simulink model "my_gm_HDLModulatorFull"  (R2024a)
settings: Solver=FixedStepDiscrete  StartTime=0.0  StopTime=stopTime  RelTol=1e-3
values from neighbouring files (symbols this model uses):
  dataSymbols = [ ... (first row only)    [testModulatorFull.m]
undefined symbols (not defined in the file or in its folder): fPHY, fs, interpolatorFilter, numDataCarriers
libraries: dspsigops x56, hdlmdlgenlib x56, hdlsllib x8, dspsrcs4 x4, commdigbbndam3 x2, whdlutilities x1, commdigbbndpm3 x1, dsphdlsigops2 x1, dsphdlfiltering2 x1, whdlmod x1, HDL_ieee_8021513 x1
(part 1 of 2)
settings Model: SimulationMode=accelerator  Creator=cotti  LastModifiedBy=cotti
settings OptimizationCC: BlockReduction=off  ConditionallyExecuteInputs=off  DefaultParameterBehavior=Inlined  InheritOutputTypeSmallerThanSingle=on
settings DebuggingCC: AlgebraicLoopMsg=error  ArtificialAlgebraicLoopMsg=none  InheritedTsInSrcMsg=none  SingleTaskRateTransMsg=error  UnconnectedInputMsg=warning  UnconnectedOutputMsg=warning  UnconnectedLineMsg=warning
settings HardwareCC: ProdBitPerPointer=32  ProdBitPerSizeT=32  ProdBitPerPtrDiffT=32  ProdLargestAtomicFloat=None  ProdIntDivRoundTo=Undefined  ProdEndianess=Unspecified  ProdWordSize=32  ProdHWDeviceType=ASIC/FPGA->ASIC/FPGA  TargetBitPerLong=64  TargetBitPerPointer=64  TargetBitPerSizeT=64  TargetBitPerPtrDiffT=64  TargetLongLongMode=on  TargetIntDivRoundTo=Zero  TargetEndianess=LittleEndian  TargetWordSize=64  TargetHWDeviceType=Custom Processor->MATLAB Host Computer  ProdEqTarget=off

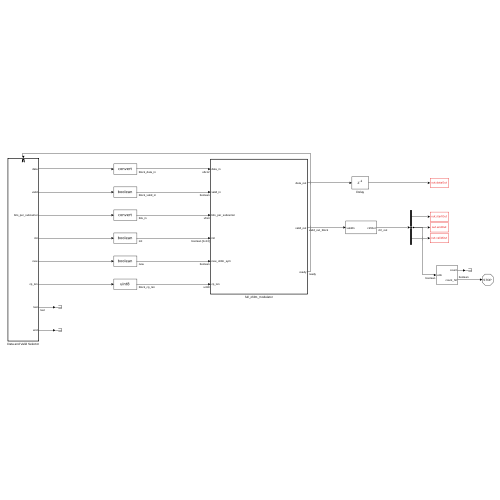
[thumbnail: Simulink's stored preview of the top-level diagram]
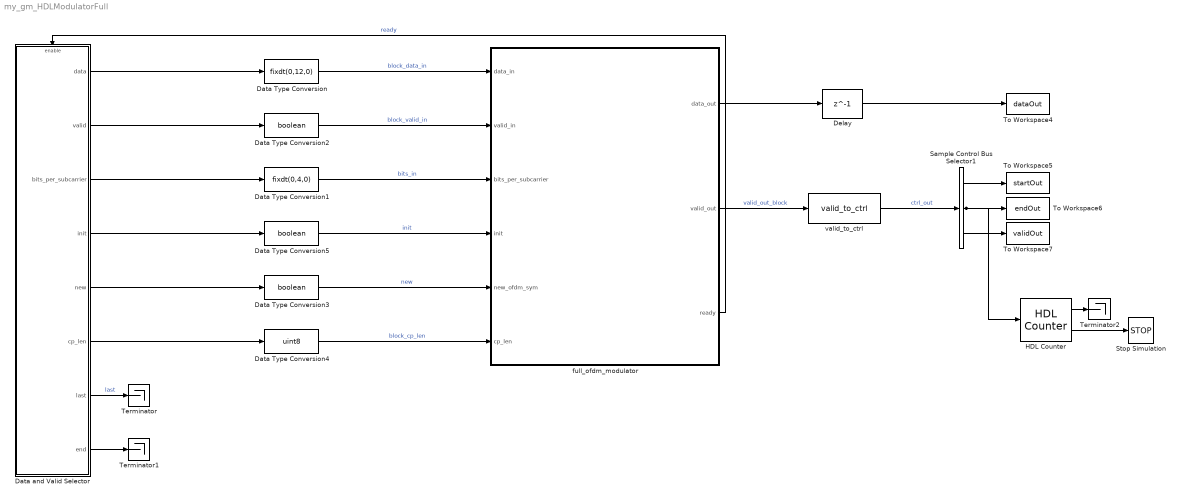
== system my_gm_HDLModulatorFull ==
  Data Type Conversion : DataTypeConversion  OutDataTypeStr=fixdt(0,12,0)  SaturateOnIntegerOverflow=off  RndMeth=Floor  LockScale=on
  Data Type Conversion1 : DataTypeConversion  OutDataTypeStr=fixdt(0,4,0)  SaturateOnIntegerOverflow=off  RndMeth=Floor  LockScale=on
  Data Type Conversion2 : DataTypeConversion  OutDataTypeStr=boolean  SaturateOnIntegerOverflow=off  RndMeth=Floor  LockScale=on
  Data Type Conversion3 : DataTypeConversion  OutDataTypeStr=boolean  SaturateOnIntegerOverflow=off  RndMeth=Floor  LockScale=on
  Data Type Conversion4 : DataTypeConversion  OutDataTypeStr=uint8  SaturateOnIntegerOverflow=off  RndMeth=Floor  LockScale=on
  Data Type Conversion5 : DataTypeConversion  OutDataTypeStr=boolean  SaturateOnIntegerOverflow=off  RndMeth=Floor  LockScale=on
  Data and Valid Selector : Subsystem  TreatAsAtomicUnit=on
  Delay : Delay  DelayLength=1  InitialCondition=0  UseCircularBuffer=on
  HDL Counter : hdlsllib/Sources/HDL Counter  CountType=Count limited  CountInit=0  CountStep=1  CountMax=numberOfRepetitions  CountFromType=Initial value  CountFrom=0  CountResetPort=off  CountLoadPort=off  CountEnbPort=on  CountDirPort=off  CountHitOutputPort=on  CountDataType=Unsigned  CountWordLen=8  CountFracLen=0  CountSampTime=1
  Sample Control Bus Selector1 : whdlutilities/Sample Control Bus Selector  OutputSignals=start,end,valid
  Stop Simulation : Stop
  Terminator : Terminator
  Terminator1 : Terminator
  Terminator2 : Terminator
  To Workspace4 : ToWorkspace  VariableName=dataOut  SampleTime=1/fs
      settings: Save2DSignal=2-D array (concatenate along first dimension)
  To Workspace5 : ToWorkspace  VariableName=startOut  SampleTime=1/fs
      settings: Save2DSignal=2-D array (concatenate along first dimension)
  To Workspace6 : ToWorkspace  VariableName=endOut  SampleTime=1/fs
      settings: Save2DSignal=2-D array (concatenate along first dimension)
  To Workspace7 : ToWorkspace  VariableName=validOut  SampleTime=1/fs
      settings: Save2DSignal=2-D array (concatenate along first dimension)
  full_ofdm_modulator : Subsystem  TreatAsAtomicUnit=on
  valid_to_ctrl : HDL_ieee_8021513/valid_to_ctrl  SystemSampleTime=-1  VariantActivationTime=update diagram  AllowFlexibleInterface=on  Latency=0  AutoFrameSizeCalculation=off
      settings: SourceProductName=HDL IEEE 8021513
  wires:
  HDL Counter/2 -> Stop Simulation/1
  HDL Counter/1 -> Terminator2/1
  Delay/1 -> To Workspace4/1
  full_ofdm_modulator/3(ready) -> Data and Valid Selector/Enable  "ready"
  Data Type Conversion5/1 -> full_ofdm_modulator/4(init)  "init"
  Data Type Conversion3/1 -> full_ofdm_modulator/5(new_ofdm_sym)  "new"
  Data and Valid Selector/7(last) -> Terminator/1  "last"
  Data and Valid Selector/5(new) -> Data Type Conversion3/1
  Data and Valid Selector/3(bits_per_subcarrier) -> Data Type Conversion1/1
  Data and Valid Selector/1(data) -> Data Type Conversion/1
  Data Type Conversion/1 -> full_ofdm_modulator/1(data_in)  "block_data_in"
  Data and Valid Selector/2(valid) -> Data Type Conversion2/1
  Data and Valid Selector/4(init) -> Data Type Conversion5/1
  Data and Valid Selector/6(cp_len) -> Data Type Conversion4/1
  Data Type Conversion4/1 -> full_ofdm_modulator/6(cp_len)  "block_cp_len"
  Data Type Conversion2/1 -> full_ofdm_modulator/2(valid_in)  "block_valid_in"
  Data and Valid Selector/8(end) -> Terminator1/1
  Data Type Conversion1/1 -> full_ofdm_modulator/3(bits_per_subcarrier)  "bits_in"
  Sample Control Bus Selector1/2 -> To Workspace6/1, HDL Counter/1
  Sample Control Bus Selector1/1 -> To Workspace5/1
  valid_to_ctrl/1 -> Sample Control Bus Selector1/1  "ctrl_out"
  Sample Control Bus Selector1/3 -> To Workspace7/1
  full_ofdm_modulator/1(data_out) -> Delay/1
  full_ofdm_modulator/2(valid_out) -> valid_to_ctrl/1  "valid_out_block"

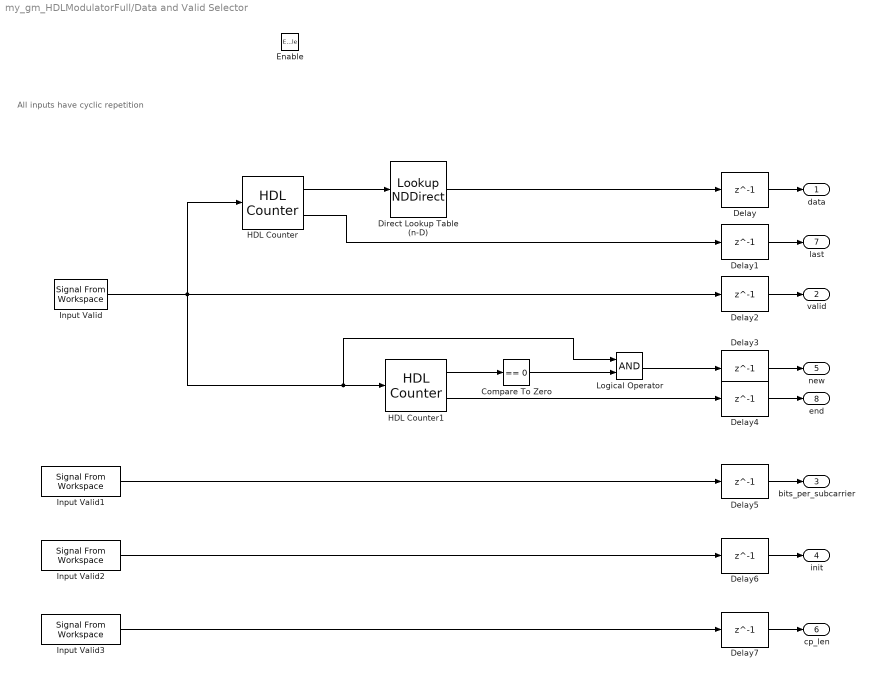
== system my_gm_HDLModulatorFull/Data and Valid Selector ==
  note: All inputs have cyclic repetition
  Enable : EnablePort
  Compare To Zero : hdlsllib/Logic and Bit Operations/Compare To Zero  relop===  OutDataTypeStr=boolean
  Delay{,1..7} (8 alike) : Delay  DelayLength=1  InitialCondition=0  UseCircularBuffer=on
  Direct Lookup Table (n-D) : LookupNDDirect  NumberOfTableDimensions=1  Table=dataSymbols  DiagnosticForOutOfRangeInput=Error  TableDataTypeStr=fixdt(0,12,0)
  HDL Counter : hdlsllib/Sources/HDL Counter  CountType=Count limited  CountInit=0  CountStep=1  CountMax=length(dataSymbols) -1  CountFromType=Initial value  CountFrom=0  CountResetPort=off  CountLoadPort=off  CountEnbPort=on  CountDirPort=off  CountHitOutputPort=on  CountDataType=Unsigned  CountWordLen=nextpow2(length(dataSymbols))  CountFracLen=0  CountSampTime=1
  HDL Counter1 : hdlsllib/Sources/HDL Counter  CountType=Count limited  CountInit=0  CountStep=1  CountMax=numDataCarriers-1  CountFromType=Initial value  CountFrom=0  CountResetPort=off  CountLoadPort=off  CountEnbPort=on  CountDirPort=off  CountHitOutputPort=on  CountDataType=Unsigned  CountWordLen=nextpow2(numDataCarriers)  CountFracLen=0  CountSampTime=1
  Input Valid : dspsrcs4/Signal From Workspace  X=validIn  Ts=1/fPHY  nsamps=1  OutputAfterFinalValue=Cyclic repetition  ignoreOrWarnInputAndFrameLengths=off  OutputFrames=off
  Input Valid1 : dspsrcs4/Signal From Workspace  X=bitsPerSubcarrier  Ts=1/fPHY  nsamps=1  OutputAfterFinalValue=Cyclic repetition  ignoreOrWarnInputAndFrameLengths=off  OutputFrames=off
  Input Valid2 : dspsrcs4/Signal From Workspace  X=init  Ts=1/fPHY  nsamps=1  OutputAfterFinalValue=Cyclic repetition  ignoreOrWarnInputAndFrameLengths=off  OutputFrames=off
  Input Valid3 : dspsrcs4/Signal From Workspace  X=cpLen  Ts=1/fPHY  nsamps=1  OutputAfterFinalValue=Cyclic repetition  ignoreOrWarnInputAndFrameLengths=off  OutputFrames=off
  Logical Operator : Logic  AllPortsSameDT=off  OutDataTypeStr=boolean
  data : Outport  InitialOutput=0  VectorParamsAs1DForOutWhenUnconnected=off
  valid : Outport  Port=2  InitialOutput=0  VectorParamsAs1DForOutWhenUnconnected=off
  bits_per_subcarrier : Outport  Port=3  VectorParamsAs1DForOutWhenUnconnected=off
  init : Outport  Port=4  VectorParamsAs1DForOutWhenUnconnected=off
  new : Outport  Port=5  VectorParamsAs1DForOutWhenUnconnected=off
  cp_len : Outport  Port=6  VectorParamsAs1DForOutWhenUnconnected=off
  last : Outport  Port=7  VectorParamsAs1DForOutWhenUnconnected=off
  end : Outport  Port=8  VectorParamsAs1DForOutWhenUnconnected=off
  wires:
  Delay7/1 -> cp_len/1
  Delay6/1 -> init/1
  Delay5/1 -> bits_per_subcarrier/1
  Delay4/1 -> end/1
  Delay3/1 -> new/1
  Delay2/1 -> valid/1
  Delay1/1 -> last/1
  Delay/1 -> data/1
  Input Valid1/1 -> Delay5/1
  Input Valid2/1 -> Delay6/1
  Input Valid3/1 -> Delay7/1
  Input Valid/1 -> HDL Counter1/1, Logical Operator/1, Delay2/1, HDL Counter/1
  HDL Counter1/2 -> Delay4/1
  Logical Operator/1 -> Delay3/1
  Compare To Zero/1 -> Logical Operator/2
  HDL Counter1/1 -> Compare To Zero/1
  HDL Counter/2 -> Delay1/1
  Direct Lookup Table (n-D)/1 -> Delay/1
  HDL Counter/1 -> Direct Lookup Table (n-D)/1

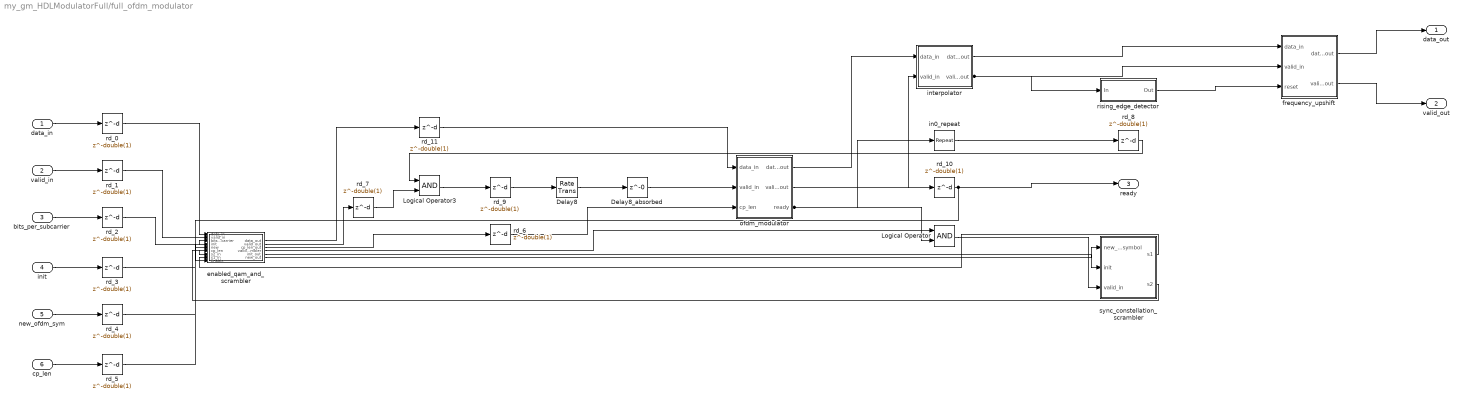
== system my_gm_HDLModulatorFull/full_ofdm_modulator ==
  data_in : Inport  OutDataTypeStr=fixdt(0, 12, 0)  PortDimensions=1  SampleTime=2e-08
  valid_in : Inport  Port=2  OutDataTypeStr=boolean  PortDimensions=1  SampleTime=2e-08
  bits_per_subcarrier : Inport  Port=3  OutDataTypeStr=fixdt(0, 4, 0)  PortDimensions=1  SampleTime=2e-08
  init : Inport  Port=4  OutDataTypeStr=boolean  PortDimensions=[1 13]  SampleTime=2e-08
  new_ofdm_sym : Inport  Port=5  OutDataTypeStr=boolean  PortDimensions=1  SampleTime=2e-08
  cp_len : Inport  Port=6  OutDataTypeStr=uint8  PortDimensions=1  SampleTime=2e-08
  Delay8 : RateTransition  OutPortSampleTimeOpt=Multiple of input port sample time  OutPortSampleTimeMultiple=2
  Delay8_absorbed : Delay  DelayLength=0
  Logical Operator : Logic  AllPortsSameDT=off  OutDataTypeStr=boolean  SampleTime=2e-08
  Logical Operator3 : Logic  AllPortsSameDT=off  OutDataTypeStr=boolean  SampleTime=1e-08
  enabled_qam_and_scrambler : Subsystem
  frequency_upshift : Subsystem
  in0_repeat : dspsigops/Repeat  FactorSource=Dialog parameter  N=double(2)  Nmax=16  RateOptions=Allow multirate processing  ic=0  mode=Unused parameter value
  interpolator : Subsystem
  ofdm_modulator : Subsystem
  rd_{0..6,10..11} (9 alike) : Delay  DelayLength=double(1)  InitialCondition=0  SampleTime=2e-08
  rd_7 : Delay  DelayLength=double(1)  InitialCondition=0  SampleTime=1e-08
  rd_8 : Delay  DelayLength=double(1)  InitialCondition=0  SampleTime=1e-08
  rd_9 : Delay  DelayLength=double(1)  InitialCondition=0  SampleTime=1e-08
  rising_edge_detector : Subsystem
  sync_constellation_scrambler : Subsystem
  data_out : Outport  SampleTime=1e-08  VectorParamsAs1DForOutWhenUnconnected=off
  valid_out : Outport  Port=2  SampleTime=1e-08  VectorParamsAs1DForOutWhenUnconnected=off
  ready : Outport  Port=3  SampleTime=2e-08  VectorParamsAs1DForOutWhenUnconnected=off
  wires:
  data_in/1 -> rd_0/1
  valid_in/1 -> rd_1/1
  bits_per_subcarrier/1 -> rd_2/1
  init/1 -> rd_3/1
  new_ofdm_sym/1 -> rd_4/1
  cp_len/1 -> rd_5/1
  frequency_upshift/1(data_out) -> data_out/1
  frequency_upshift/2(valid_out) -> valid_out/1
  interpolator/1(data_out) -> frequency_upshift/1(data_in)
  interpolator/2(valid_out) -> frequency_upshift/2(valid_in), rising_edge_detector/1(In)
  ofdm_modulator/1(data_out) -> interpolator/1(data_in)
  ofdm_modulator/2(valid_out) -> interpolator/2(valid_in)
  rising_edge_detector/1(Out) -> frequency_upshift/3(reset)
  sync_constellation_scrambler/1(s1) -> enabled_qam_and_scrambler/8(s1_in)
  enabled_qam_and_scrambler/1(data_out) -> rd_11/1
  enabled_qam_and_scrambler/3(cp_len_out) -> rd_6/1
  sync_constellation_scrambler/2(s2) -> enabled_qam_and_scrambler/7(s2_in)
  enabled_qam_and_scrambler/2(valid_out) -> rd_7/1
  enabled_qam_and_scrambler/4(valid_scrambler) -> Logical Operator/1
  enabled_qam_and_scrambler/5(init_out) -> sync_constellation_scrambler/2(init)
  enabled_qam_and_scrambler/6(new_out) -> sync_constellation_scrambler/1(new_ofdm_symbol)
  ofdm_modulator/3(ready) -> Logical Operator/2, in0_repeat/1, rd_10/1
  in0_repeat/1 -> rd_8/1
  Delay8/1 -> Delay8_absorbed/1
  Delay8_absorbed/1 -> ofdm_modulator/2(valid_in)
  Logical Operator/1 -> sync_constellation_scrambler/3(valid_in)
  Logical Operator3/1 -> rd_9/1
  rd_1/1 -> enabled_qam_and_scrambler/2(valid_in)
  rd_2/1 -> enabled_qam_and_scrambler/3(bits_per_subcarrier)
  rd_3/1 -> enabled_qam_and_scrambler/4(init)
  rd_4/1 -> enabled_qam_and_scrambler/5(new)
  rd_5/1 -> enabled_qam_and_scrambler/6(cp_len)
  rd_0/1 -> enabled_qam_and_scrambler/1(data_in)
  rd_8/1 -> Logical Operator3/1
  rd_9/1 -> Delay8/1
  rd_7/1 -> Logical Operator3/2
  rd_11/1 -> ofdm_modulator/1(data_in)
  rd_6/1 -> ofdm_modulator/3(cp_len)
  rd_10/1 -> enabled_qam_and_scrambler/9(Enable), ready/1

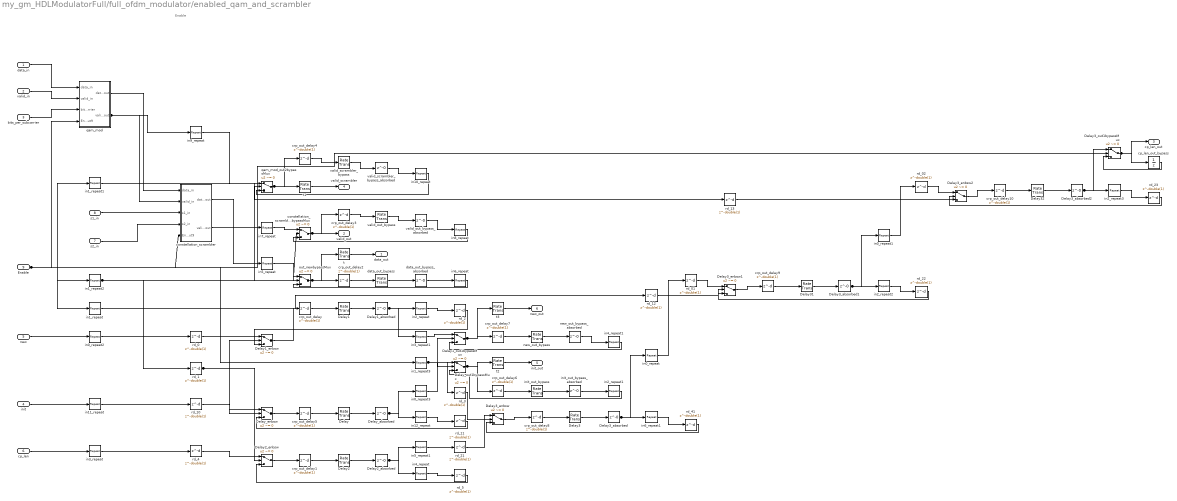
== system my_gm_HDLModulatorFull/full_ofdm_modulator/enabled_qam_and_scrambler ==
  note: Enable
  data_in : Inport  OutDataTypeStr=fixdt(0, 12, 0)  PortDimensions=1  SampleTime=2e-08
  valid_in : Inport  Port=2  OutDataTypeStr=boolean  PortDimensions=1  SampleTime=2e-08
  bits_per_subcarrier : Inport  Port=3  OutDataTypeStr=fixdt(0, 4, 0)  PortDimensions=1  SampleTime=2e-08
  init : Inport  Port=4  OutDataTypeStr=boolean  PortDimensions=[1 13]  SampleTime=2e-08
  new : Inport  Port=5  OutDataTypeStr=boolean  PortDimensions=1  SampleTime=2e-08
  cp_len : Inport  Port=6  OutDataTypeStr=uint8  PortDimensions=1  SampleTime=2e-08
  s2_in : Inport  Port=7  OutDataTypeStr=boolean  PortDimensions=1  SampleTime=2e-08
  s1_in : Inport  Port=8  OutDataTypeStr=boolean  PortDimensions=1  SampleTime=2e-08
  Enable : Inport  Port=9  OutDataTypeStr=boolean  SampleTime=2e-08
  Delay{,1..3,31..32} (6 alike) : RateTransition  OutPortSampleTimeOpt=Multiple of input port sample time  OutPortSampleTimeMultiple=2
  Delay1_absorbed : Delay  DelayLength=0
  Delay1_enbsw : Switch  Criteria=u2 ~= 0  Threshold=double(0)  OutDataTypeStr=boolean  SampleTime=1e-08  SaturateOnIntegerOverflow=off  InputSameDT=off
  Delay1_out1bypassMux : Switch  Criteria=u2 ~= 0  Threshold=double(0)  OutDataTypeStr=boolean  SampleTime=1e-08  SaturateOnIntegerOverflow=off  InputSameDT=off
  Delay2_absorbed : Delay  DelayLength=0
  Delay2_enbsw : Switch  Criteria=u2 ~= 0  Threshold=double(0)  OutDataTypeStr=uint8  SampleTime=1e-08  SaturateOnIntegerOverflow=off  InputSameDT=off
  Delay3_absorbed : Delay  DelayLength=0
  Delay3_absorbed1 : Delay  DelayLength=0
  Delay3_absorbed2 : Delay  DelayLength=0
  Delay3_enbsw : Switch  Criteria=u2 ~= 0  Threshold=double(0)  OutDataTypeStr=uint8  SampleTime=1e-08  SaturateOnIntegerOverflow=off  InputSameDT=off
  Delay3_enbsw1 : Switch  Criteria=u2 ~= 0  Threshold=double(0)  OutDataTypeStr=uint8  SampleTime=1e-08  SaturateOnIntegerOverflow=off  InputSameDT=off
  Delay3_enbsw2 : Switch  Criteria=u2 ~= 0  Threshold=double(0)  OutDataTypeStr=uint8  SampleTime=1e-08  SaturateOnIntegerOverflow=off  InputSameDT=off
  Delay3_out1bypassMux : Switch  Criteria=u2 ~= 0  Threshold=double(0)  OutDataTypeStr=uint8  SampleTime=2e-08  SaturateOnIntegerOverflow=off  InputSameDT=off
  Delay_absorbed : Delay  DelayLength=0
  Delay_enbsw : Switch  Criteria=u2 ~= 0  Threshold=double(0)  OutDataTypeStr=boolean  SampleTime=1e-08  SaturateOnIntegerOverflow=off  InputSameDT=off
  Delay_out1bypassMux : Switch  Criteria=u2 ~= 0  Threshold=double(0)  OutDataTypeStr=boolean  SampleTime=1e-08  SaturateOnIntegerOverflow=off  InputSameDT=off
  constellation_scrambler : Subsystem
  constellation_scrambler_out2bypassMux : Switch  Criteria=u2 ~= 0  Threshold=double(0)  OutDataTypeStr=boolean  SampleTime=1e-08  SaturateOnIntegerOverflow=off  InputSameDT=off
  cp_len_out_bypass : UnitDelay  SampleTime=2e-08
  crp_out_delay{,1..10} (11 alike) : Delay  DelayLength=double(1)  InitialCondition=0
  data_out_bypass : RateTransition  OutPortSampleTimeOpt=Multiple of input port sample time  OutPortSampleTimeMultiple=2
  data_out_bypass_absorbed : Delay  DelayLength=0
  in0_repeat{,1..3} (4 alike) : dspsigops/Repeat  FactorSource=Dialog parameter  N=double(2)  Nmax=16  RateOptions=Allow multirate processing  ic=0  mode=Unused parameter value
  in10_repeat : dspsigops/Repeat  FactorSource=Dialog parameter  N=double(2)  Nmax=16  RateOptions=Allow multirate processing  ic=0  mode=Unused parameter value
  in11_repeat : dspsigops/Repeat  FactorSource=Dialog parameter  N=double(2)  Nmax=16  RateOptions=Allow multirate processing  ic=0  mode=Unused parameter value
  in12_repeat : dspsigops/Repeat  FactorSource=Dialog parameter  N=double(2)  Nmax=16  RateOptions=Allow multirate processing  ic=0  mode=Unused parameter value
  in1_repeat{,1..3} (4 alike) : dspsigops/Repeat  FactorSource=Dialog parameter  N=double(2)  Nmax=16  RateOptions=Allow multirate processing  ic=0  mode=Unused parameter value
  in2_repeat{,1..3} (4 alike) : dspsigops/Repeat  FactorSource=Dialog parameter  N=double(2)  Nmax=16  RateOptions=Allow multirate processing  ic=0  mode=Unused parameter value
  in3_repeat : dspsigops/Repeat  FactorSource=Dialog parameter  N=double(2)  Nmax=16  RateOptions=Allow multirate processing  ic=0  mode=Unused parameter value
  in3_repeat1 : dspsigops/Repeat  FactorSource=Dialog parameter  N=double(2)  Nmax=16  RateOptions=Allow multirate processing  ic=0  mode=Unused parameter value
  in4_repeat : dspsigops/Repeat  FactorSource=Dialog parameter  N=double(2)  Nmax=16  RateOptions=Allow multirate processing  ic=0  mode=Unused parameter value
  in4_repeat1 : dspsigops/Repeat  FactorSource=Dialog parameter  N=double(2)  Nmax=16  RateOptions=Allow multirate processing  ic=0  mode=Unused parameter value
  in5_repeat : dspsigops/Repeat  FactorSource=Dialog parameter  N=double(2)  Nmax=16  RateOptions=Allow multirate processing  ic=0  mode=Unused parameter value
  in5_repeat1 : dspsigops/Repeat  FactorSource=Dialog parameter  N=double(2)  Nmax=16  RateOptions=Allow multirate processing  ic=0  mode=Unused parameter value
  in6_repeat : dspsigops/Repeat  FactorSource=Dialog parameter  N=double(2)  Nmax=16  RateOptions=Allow multirate processing  ic=0  mode=Unused parameter value
  in6_repeat1 : dspsigops/Repeat  FactorSource=Dialog parameter  N=double(2)  Nmax=16  RateOptions=Allow multirate processing  ic=0  mode=Unused parameter value
  in7_repeat : dspsigops/Repeat  FactorSource=Dialog parameter  N=double(2)  Nmax=16  RateOptions=Allow multirate processing  ic=0  mode=Unused parameter value
  in8_repeat : dspsigops/Repeat  FactorSource=Dialog parameter  N=double(2)  Nmax=16  RateOptions=Allow multirate processing  ic=0  mode=Unused parameter value
  in9_repeat : dspsigops/Repeat  FactorSource=Dialog parameter  N=double(2)  Nmax=16  RateOptions=Allow multirate processing  ic=0  mode=Unused parameter value
  init_out_bypass : RateTransition  OutPortSampleTimeOpt=Multiple of input port sample time  OutPortSampleTimeMultiple=2
  init_out_bypass_absorbed : Delay  DelayLength=0
  new_out_bypass : RateTransition  OutPortSampleTimeOpt=Multiple of input port sample time  OutPortSampleTimeMultiple=2
  new_out_bypass_absorbed : Delay  DelayLength=0
  out_newbypassMux : Switch  Criteria=u2 ~= 0  Threshold=double(0)  OutDataTypeStr=fixdt(1, 16, 14)  SampleTime=1e-08  SaturateOnIntegerOverflow=off  InputSameDT=off
  qam_mod : Subsystem
  qam_mod_out2bypassMux : Switch  Criteria=u2 ~= 0  Threshold=double(0)  OutDataTypeStr=boolean  SampleTime=1e-08  SaturateOnIntegerOverflow=off  InputSameDT=off
  rd_{0..5,10..13,21..23,41} (14 alike) : Delay  DelayLength=double(1)  InitialCondition=0
  rd_01 : Delay  DelayLength=double(1)  InitialCondition=0
  rd_02 : Delay  DelayLength=double(1)  InitialCondition=0
  t{,1..3} (4 alike) : RateTransition  OutPortSampleTimeOpt=Multiple of input port sample time  OutPortSampleTimeMultiple=2
  valid_out_bypass : RateTransition  OutPortSampleTimeOpt=Multiple of input port sample time  OutPortSampleTimeMultiple=2
  valid_out_bypass_absorbed : Delay  DelayLength=0
  valid_scrambler_bypass : RateTransition  OutPortSampleTimeOpt=Multiple of input port sample time  OutPortSampleTimeMultiple=2
  valid_scrambler_bypass_absorbed : Delay  DelayLength=0
  data_out : Outport  SampleTime=2e-08  InitialOutput=0  VectorParamsAs1DForOutWhenUnconnected=off
  valid_out : Outport  Port=2  SampleTime=1e-08  InitialOutput=0  VectorParamsAs1DForOutWhenUnconnected=off
  cp_len_out : Outport  Port=3  SampleTime=2e-08  InitialOutput=0  VectorParamsAs1DForOutWhenUnconnected=off
  valid_scrambler : Outport  Port=4  SampleTime=2e-08  InitialOutput=0  VectorParamsAs1DForOutWhenUnconnected=off
  init_out : Outport  Port=5  SampleTime=2e-08  InitialOutput=0  VectorParamsAs1DForOutWhenUnconnected=off
  new_out : Outport  Port=6  SampleTime=2e-08  InitialOutput=0  VectorParamsAs1DForOutWhenUnconnected=off
  wires:
  Enable/1 -> qam_mod/4(Enable_out9), constellation_scrambler/5(Enable_out9), in1_repeat2/1, in1_repeat/1, in1_repeat1/1, in1_repeat3/1, Delay3_out1bypassMux/2
  data_in/1 -> qam_mod/1(data_in)
  valid_in/1 -> qam_mod/2(valid_in)
  bits_per_subcarrier/1 -> qam_mod/3(bits_per_subcarrier)
  init/1 -> in11_repeat/1
  new/1 -> in0_repeat2/1
  cp_len/1 -> in3_repeat/1
  s2_in/1 -> constellation_scrambler/4(s2_in)
  s1_in/1 -> constellation_scrambler/3(s1_in)
  constellation_scrambler/1(data_out) -> in5_repeat/1
  constellation_scrambler/2(valid_out) -> in7_repeat/1
  qam_mod/1(data_out) -> constellation_scrambler/1(data_in)
  qam_mod/2(valid_out) -> constellation_scrambler/2(valid_in), in9_repeat/1
  t/1 -> data_out/1
  Delay3_out1bypassMux/1 -> cp_len_out/1, cp_len_out_bypass/1
  t1/1 -> valid_scrambler/1
  t2/1 -> init_out/1
  t3/1 -> new_out/1
  constellation_scrambler_out2bypassMux/1 -> valid_out/1, crp_out_delay3/1
  Delay1_absorbed/1 -> in3_repeat1/1, in2_repeat/1
  Delay2_absorbed/1 -> in5_repeat1/1, in4_repeat/1
  Delay_absorbed/1 -> in0_repeat3/1, in12_repeat/1
  Delay3_absorbed1/1 -> in0_repeat1/1, in2_repeat2/1
  Delay3_absorbed2/1 -> in2_repeat3/1, Delay3_out1bypassMux/1
  Delay3_absorbed/1 -> in0_repeat/1, in6_repeat1/1
  in0_repeat2/1 -> rd_0/1
  in1_repeat2/1 -> qam_mod_out2bypassMux/2, constellation_scrambler_out2bypassMux/2, out_newbypassMux/2, rd_1/1
  in3_repeat/1 -> rd_4/1
  in5_repeat/1 -> out_newbypassMux/1
  in7_repeat/1 -> constellation_scrambler_out2bypassMux/1
  in9_repeat/1 -> qam_mod_out2bypassMux/1
  in11_repeat/1 -> rd_10/1
  out_newbypassMux/1 -> t/1, crp_out_delay2/1
  qam_mod_out2bypassMux/1 -> t1/1, crp_out_delay4/1
  in0_repeat/1 -> rd_01/1
  in1_repeat/1 -> rd_12/1
  in0_repeat1/1 -> rd_02/1
  in1_repeat1/1 -> rd_13/1
  in0_repeat3/1 -> Delay_out1bypassMux/1
  in1_repeat3/1 -> rd_3/1, Delay_out1bypassMux/2, Delay1_out1bypassMux/2
  in3_repeat1/1 -> Delay1_out1bypassMux/1
  in5_repeat1/1 -> rd_21/1
  Delay_out1bypassMux/1 -> t2/1, crp_out_delay6/1
  Delay1_out1bypassMux/1 -> t3/1, crp_out_delay7/1
  in12_repeat/1 -> rd_11/1
  valid_scrambler_bypass/1 -> valid_scrambler_bypass_absorbed/1
  valid_scrambler_bypass_absorbed/1 -> in10_repeat/1
  in10_repeat/1 -> qam_mod_out2bypassMux/3
  valid_out_bypass/1 -> valid_out_bypass_absorbed/1
  valid_out_bypass_absorbed/1 -> in8_repeat/1
  in8_repeat/1 -> constellation_scrambler_out2bypassMux/3
  data_out_bypass/1 -> data_out_bypass_absorbed/1
  data_out_bypass_absorbed/1 -> in6_repeat/1
  in6_repeat/1 -> out_newbypassMux/3
  Delay2/1 -> Delay2_absorbed/1
  in4_repeat/1 -> rd_5/1
  Delay1/1 -> Delay1_absorbed/1
  in2_repeat/1 -> rd_2/1
  crp_out_delay/1 -> Delay1/1
  crp_out_delay1/1 -> Delay2/1
  crp_out_delay2/1 -> data_out_bypass/1
  crp_out_delay3/1 -> valid_out_bypass/1
  crp_out_delay4/1 -> valid_scrambler_bypass/1
  crp_out_delay5/1 -> Delay/1
  Delay/1 -> Delay_absorbed/1
  Delay3/1 -> Delay3_absorbed/1
  in6_repeat1/1 -> rd_41/1
  new_out_bypass/1 -> new_out_bypass_absorbed/1
  new_out_bypass_absorbed/1 -> in4_repeat1/1
  in4_repeat1/1 -> Delay1_out1bypassMux/3
  init_out_bypass/1 -> init_out_bypass_absorbed/1
  init_out_bypass_absorbed/1 -> in2_repeat1/1
  in2_repeat1/1 -> Delay_out1bypassMux/3
  crp_out_delay6/1 -> init_out_bypass/1
  crp_out_delay7/1 -> new_out_bypass/1
  crp_out_delay8/1 -> Delay3/1
  in2_repeat2/1 -> rd_22/1
  crp_out_delay9/1 -> Delay31/1
  Delay31/1 -> Delay3_absorbed1/1
  in2_repeat3/1 -> rd_23/1
  crp_out_delay10/1 -> Delay32/1
  Delay32/1 -> Delay3_absorbed2/1
  cp_len_out_bypass/1 -> Delay3_out1bypassMux/3
  Delay1_enbsw/1 -> crp_out_delay/1
  Delay2_enbsw/1 -> crp_out_delay1/1
  Delay_enbsw/1 -> crp_out_delay5/1
  rd_10/1 -> Delay_enbsw/1
  rd_11/1 -> Delay_enbsw/3
  rd_0/1 -> Delay1_enbsw/1
  rd_2/1 -> Delay1_enbsw/3
  rd_4/1 -> Delay2_enbsw/1
  rd_5/1 -> Delay2_enbsw/3
  rd_1/1 -> Delay2_enbsw/2, Delay1_enbsw/2, Delay_enbsw/2
  Delay3_enbsw/1 -> crp_out_delay8/1
  rd_3/1 -> Delay3_enbsw/2
  rd_21/1 -> Delay3_enbsw/1
  rd_41/1 -> Delay3_enbsw/3
  Delay3_enbsw1/1 -> crp_out_delay9/1
  rd_01/1 -> Delay3_enbsw1/1
  rd_12/1 -> Delay3_enbsw1/2
  rd_22/1 -> Delay3_enbsw1/3
  Delay3_enbsw2/1 -> crp_out_delay10/1
  rd_02/1 -> Delay3_enbsw2/1
  rd_13/1 -> Delay3_enbsw2/2
  rd_23/1 -> Delay3_enbsw2/3

== system my_gm_HDLModulatorFull/full_ofdm_modulator/frequency_upshift ==
  data_in : Inport  OutDataTypeStr=fixdt(1, 16, 14)  SampleTime=1e-08
      settings: SignalType=complex
  valid_in : Inport  Port=2  OutDataTypeStr=boolean  SampleTime=1e-08
  reset : Inport  Port=3  OutDataTypeStr=boolean  SampleTime=1e-08
  Mixer : Subsystem
  NCO : dsphdlsigops2/NCO  PhaseIncrementSource=Property  PhaseIncrement=ncoUpshifterPhaseIncrement  PhaseOffsetSource=Property  PhaseOffset=0  DitherSource=None  NumDitherBits=1  SamplesPerFrame=1  LUTCompress=off  ResetAction=on  Waveform=Complex exponential  PhasePort=off  SimulateUsing=Code generation  AccumulatorWL=ncoUpshifterWordLength  PhaseQuantization=off  NumQuantizerAccumulatorBits=6  OutputDataType=Binary point scaling  OutputWL=16  OutputFL=14
  rd_0 : Delay  DelayLength=double(1)  InitialCondition=0  SampleTime=1e-08
  rd_1 : Delay  DelayLength=double(4)  InitialCondition=0  SampleTime=1e-08
  data_out : Outport  SampleTime=1e-08
  valid_out : Outport  Port=2  SampleTime=1e-08
  wires:
  data_in/1 -> Mixer/1(dataIn)
  valid_in/1 -> rd_0/1
  reset/1 -> NCO/1
  Mixer/1(mixedOut) -> data_out/1
  NCO/1 -> Mixer/2(ncoIn)
  NCO/2 -> rd_1/1
  rd_1/1 -> valid_out/1
  rd_0/1 -> NCO/2

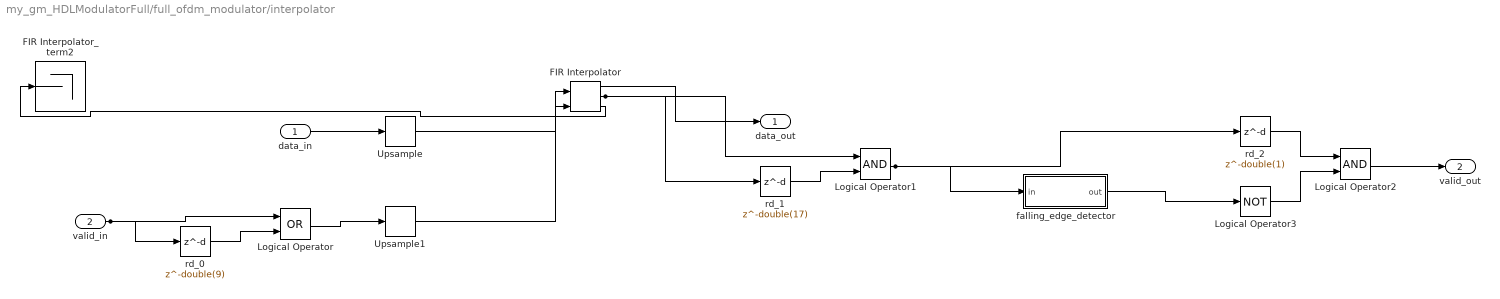
== system my_gm_HDLModulatorFull/full_ofdm_modulator/interpolator ==
  data_in : Inport  OutDataTypeStr=fixdt(1, 16, 14)  SampleTime=2e-08
      settings: SignalType=complex
  valid_in : Inport  Port=2  OutDataTypeStr=boolean  SampleTime=2e-08
  FIR Interpolator : dsphdlfiltering2/FIR Interpolator  Numerator=interpolatorFilter.Numerator  FilterStructure=Direct form systolic  InterpolationFactor=oversamplingFactor  NumCycles=oversamplingFactor  SimulateUsing=Code generation  roundingMode=Floor  overflowMode=off  CoefficientsDataTypeStr=fixdt(1,16,14)  OutputDataTypeStr=fixdt(1,16,14)  ResetInputPort=off  HDLGlobalReset=off
  FIR Interpolator_term2 : Terminator
  Logical Operator : Logic  Operator=OR  AllPortsSameDT=off  OutDataTypeStr=boolean  SampleTime=2e-08
  Logical Operator1 : Logic  AllPortsSameDT=off  OutDataTypeStr=boolean  SampleTime=1e-08
  Logical Operator2 : Logic  AllPortsSameDT=off  OutDataTypeStr=boolean  SampleTime=1e-08
  Logical Operator3 : Logic  Operator=NOT  Inputs=1  AllPortsSameDT=off  OutDataTypeStr=boolean  SampleTime=1e-08
  Upsample : dspsigops/Upsample  FactorSource=Dialog parameter  N=double(2)  Nmax=16  phase=double(0)  RateOptions=Allow multirate processing  ic=0  mode=Unused parameter value
  Upsample1 : dspsigops/Upsample  FactorSource=Dialog parameter  N=double(2)  Nmax=16  phase=double(0)  RateOptions=Allow multirate processing  ic=0  mode=Unused parameter value
  falling_edge_detector : Subsystem
  rd_0 : Delay  DelayLength=double(9)  InitialCondition=0  SampleTime=2e-08
  rd_1 : Delay  DelayLength=double(17)  InitialCondition=0  SampleTime=1e-08
  rd_2 : Delay  DelayLength=double(1)  InitialCondition=0  SampleTime=1e-08
  data_out : Outport  SampleTime=1e-08
  valid_out : Outport  Port=2  SampleTime=1e-08
  wires:
  data_in/1 -> Upsample/1
  valid_in/1 -> rd_0/1, Logical Operator/1
  FIR Interpolator/1 -> data_out/1
  FIR Interpolator/2 -> rd_1/1, Logical Operator1/1
  FIR Interpolator/3 -> FIR Interpolator_term2/1
  Logical Operator1/1 -> rd_2/1, falling_edge_detector/1(in)
  Logical Operator2/1 -> valid_out/1
  falling_edge_detector/1(out) -> Logical Operator3/1
  Upsample/1 -> FIR Interpolator/1
  Upsample1/1 -> FIR Interpolator/2
  Logical Operator3/1 -> Logical Operator2/2
  Logical Operator/1 -> Upsample1/1
  rd_2/1 -> Logical Operator2/1
  rd_1/1 -> Logical Operator1/2
  rd_0/1 -> Logical Operator/2

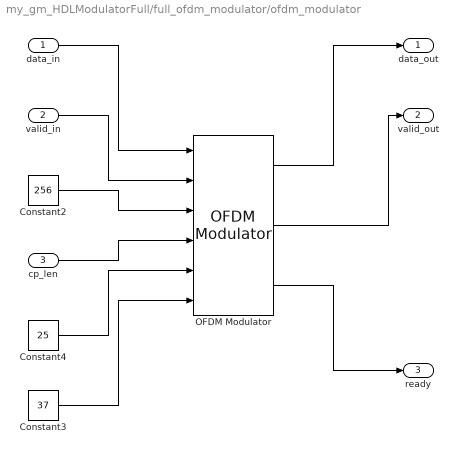
== system my_gm_HDLModulatorFull/full_ofdm_modulator/ofdm_modulator ==
  data_in : Inport  OutDataTypeStr=fixdt(1, 16, 14)  SampleTime=2e-08
      settings: SignalType=complex
  valid_in : Inport  Port=2  OutDataTypeStr=boolean  SampleTime=2e-08
  cp_len : Inport  Port=3  OutDataTypeStr=uint8  SampleTime=2e-08
  Constant2 : Constant  Value=256  OutDataTypeStr=fixdt(0, 9, 0)  SampleTime=2e-08
  Constant3 : Constant  Value=37  OutDataTypeStr=fixdt(0, 6, 0)  SampleTime=2e-08
  Constant4 : Constant  Value=25  OutDataTypeStr=fixdt(0, 6, 0)  SampleTime=2e-08
  OFDM Modulator : whdlmod/OFDM Modulator  OFDMParametersSource=Input Port  FFTLength=64  MaxFFTLength=N  CPLength=16  numLgSc=6  numRgSc=5  InsertDCNull=off  Windowing=off  WindowLength=4  MaxWindowLength=8  ResetInputPort=off  Normalize=on  RoundingMethod=Floor  SimulateUsing=Code generation
  data_out : Outport  SampleTime=2e-08
  valid_out : Outport  Port=2  SampleTime=2e-08
  ready : Outport  Port=3  SampleTime=2e-08
  wires:
  data_in/1 -> OFDM Modulator/1
  valid_in/1 -> OFDM Modulator/2
  cp_len/1 -> OFDM Modulator/4
  Constant2/1 -> OFDM Modulator/3
  Constant3/1 -> OFDM Modulator/6
  Constant4/1 -> OFDM Modulator/5
  OFDM Modulator/1 -> data_out/1
  OFDM Modulator/2 -> valid_out/1
  OFDM Modulator/3 -> ready/1

== system my_gm_HDLModulatorFull/full_ofdm_modulator/rising_edge_detector ==
  In : Inport  OutDataTypeStr=boolean  SampleTime=1e-08
  Delay2 : Delay  DelayLength=double(1)  InitialCondition=0  SampleTime=1e-08
  Logical Operator1 : Logic  AllPortsSameDT=off  OutDataTypeStr=boolean  SampleTime=1e-08
  Logical Operator2 : Logic  Operator=NOT  Inputs=1  AllPortsSameDT=off  OutDataTypeStr=boolean  SampleTime=1e-08
  Out : Outport  SampleTime=1e-08
  wires:
  In/1 -> Logical Operator1/1, Delay2/1
  Delay2/1 -> Logical Operator2/1
  Logical Operator1/1 -> Out/1
  Logical Operator2/1 -> Logical Operator1/2

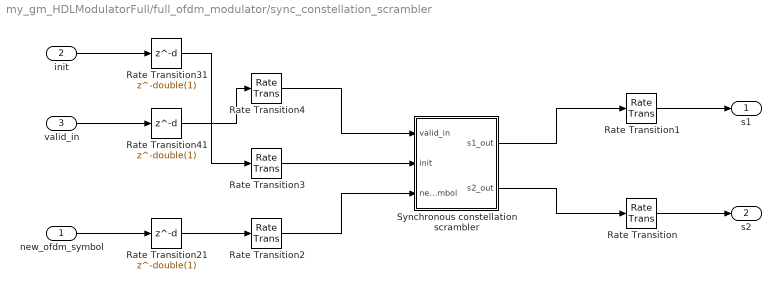
== system my_gm_HDLModulatorFull/full_ofdm_modulator/sync_constellation_scrambler ==
  new_ofdm_symbol : Inport  OutDataTypeStr=boolean  SampleTime=2e-08
  init : Inport  Port=2  OutDataTypeStr=boolean  PortDimensions=[1 13]  SampleTime=2e-08
  valid_in : Inport  Port=3  OutDataTypeStr=boolean  SampleTime=2e-08
  Rate Transition : RateTransition  InitialCondition=double(0)  OutPortSampleTimeOpt=Multiple of input port sample time  OutPortSampleTimeMultiple=2
  Rate Transition1 : RateTransition  InitialCondition=double(0)  OutPortSampleTimeOpt=Multiple of input port sample time  OutPortSampleTimeMultiple=2
  Rate Transition2 : RateTransition  Integrity=off  Deterministic=off  OutPortSampleTimeOpt=Multiple of input port sample time  OutPortSampleTimeMultiple=1/2
  Rate Transition21 : Delay  DelayLength=double(1)  InitialCondition=0  SampleTime=2e-08
  Rate Transition3 : RateTransition  Integrity=off  Deterministic=off  OutPortSampleTimeOpt=Multiple of input port sample time  OutPortSampleTimeMultiple=1/2
  Rate Transition31 : Delay  DelayLength=double(1)  InitialCondition=0  SampleTime=2e-08
  Rate Transition4 : RateTransition  Integrity=off  Deterministic=off  OutPortSampleTimeOpt=Multiple of input port sample time  OutPortSampleTimeMultiple=1/2
  Rate Transition41 : Delay  DelayLength=double(1)  InitialCondition=0  SampleTime=2e-08
  Synchronous constellation scrambler : Subsystem
  s1 : Outport  SampleTime=2e-08
  s2 : Outport  Port=2  SampleTime=2e-08
  wires:
  new_ofdm_symbol/1 -> Rate Transition21/1
  init/1 -> Rate Transition31/1
  valid_in/1 -> Rate Transition41/1
  Synchronous constellation scrambler/1(s1_out) -> Rate Transition1/1
  Synchronous constellation scrambler/2(s2_out) -> Rate Transition/1
  Rate Transition2/1 -> Synchronous constellation scrambler/3(new_ofdm_symbol)
  Rate Transition3/1 -> Synchronous constellation scrambler/2(init)
  Rate Transition4/1 -> Synchronous constellation scrambler/1(valid_in)
  Rate Transition31/1 -> Rate Transition3/1
  Rate Transition41/1 -> Rate Transition4/1
  Rate Transition21/1 -> Rate Transition2/1
  Rate Transition1/1 -> s1/1
  Rate Transition/1 -> s2/1

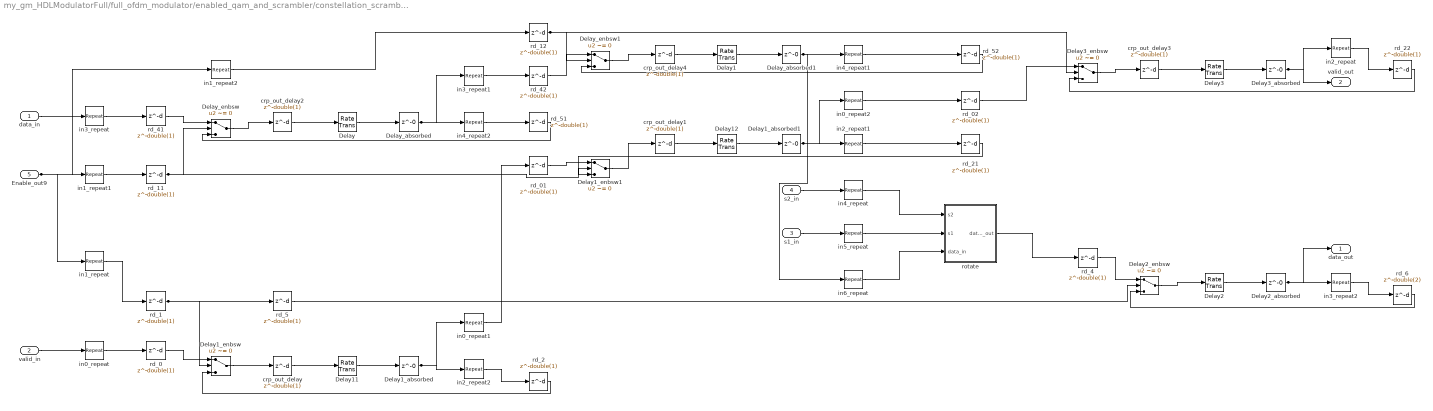
== system my_gm_HDLModulatorFull/full_ofdm_modulator/enabled_qam_and_scrambler/constellation_scrambler ==
  data_in : Inport  OutDataTypeStr=fixdt(1, 16, 14)  SampleTime=2e-08
      settings: SignalType=complex
  valid_in : Inport  Port=2  OutDataTypeStr=boolean  SampleTime=2e-08
  s1_in : Inport  Port=3  OutDataTypeStr=boolean  SampleTime=2e-08
  s2_in : Inport  Port=4  OutDataTypeStr=boolean  SampleTime=2e-08
  Enable_out9 : Inport  Port=5  OutDataTypeStr=boolean  SampleTime=2e-08
  Delay{,1..3,11..12} (6 alike) : RateTransition  OutPortSampleTimeOpt=Multiple of input port sample time  OutPortSampleTimeMultiple=2
  Delay1_absorbed : Delay  DelayLength=0
  Delay1_absorbed1 : Delay  DelayLength=0
  Delay1_enbsw : Switch  Criteria=u2 ~= 0  Threshold=double(0)  OutDataTypeStr=boolean  SampleTime=1e-08  SaturateOnIntegerOverflow=off  InputSameDT=off
  Delay1_enbsw1 : Switch  Criteria=u2 ~= 0  Threshold=double(0)  OutDataTypeStr=boolean  SampleTime=1e-08  SaturateOnIntegerOverflow=off  InputSameDT=off
  Delay2_absorbed : Delay  DelayLength=0
  Delay2_enbsw : Switch  Criteria=u2 ~= 0  Threshold=double(0)  OutDataTypeStr=fixdt(1, 16, 14)  SampleTime=1e-08  SaturateOnIntegerOverflow=off  InputSameDT=off
  Delay3_absorbed : Delay  DelayLength=0
  Delay3_enbsw : Switch  Criteria=u2 ~= 0  Threshold=double(0)  OutDataTypeStr=boolean  SampleTime=1e-08  SaturateOnIntegerOverflow=off  InputSameDT=off
  Delay_absorbed : Delay  DelayLength=0
  Delay_absorbed1 : Delay  DelayLength=0
  Delay_enbsw : Switch  Criteria=u2 ~= 0  Threshold=double(0)  OutDataTypeStr=fixdt(1, 16, 14)  SampleTime=1e-08  SaturateOnIntegerOverflow=off  InputSameDT=off
  Delay_enbsw1 : Switch  Criteria=u2 ~= 0  Threshold=double(0)  OutDataTypeStr=fixdt(1, 16, 14)  SampleTime=1e-08  SaturateOnIntegerOverflow=off  InputSameDT=off
  crp_out_delay{,1..4} (5 alike) : Delay  DelayLength=double(1)  InitialCondition=0
  in0_repeat : dspsigops/Repeat  FactorSource=Dialog parameter  N=double(2)  Nmax=16  RateOptions=Allow multirate processing  ic=0  mode=Unused parameter value
  in0_repeat1 : dspsigops/Repeat  FactorSource=Dialog parameter  N=double(2)  Nmax=16  RateOptions=Allow multirate processing  ic=0  mode=Unused parameter value
  in0_repeat2 : dspsigops/Repeat  FactorSource=Dialog parameter  N=double(2)  Nmax=16  RateOptions=Allow multirate processing  ic=0  mode=Unused parameter value
  in1_repeat : dspsigops/Repeat  FactorSource=Dialog parameter  N=double(2)  Nmax=16  RateOptions=Allow multirate processing  ic=0  mode=Unused parameter value
  in1_repeat1 : dspsigops/Repeat  FactorSource=Dialog parameter  N=double(2)  Nmax=16  RateOptions=Allow multirate processing  ic=0  mode=Unused parameter value
  in1_repeat2 : dspsigops/Repeat  FactorSource=Dialog parameter  N=double(2)  Nmax=16  RateOptions=Allow multirate processing  ic=0  mode=Unused parameter value
  in2_repeat : dspsigops/Repeat  FactorSource=Dialog parameter  N=double(2)  Nmax=16  RateOptions=Allow multirate processing  ic=0  mode=Unused parameter value
  in2_repeat1 : dspsigops/Repeat  FactorSource=Dialog parameter  N=double(2)  Nmax=16  RateOptions=Allow multirate processing  ic=0  mode=Unused parameter value
  in2_repeat2 : dspsigops/Repeat  FactorSource=Dialog parameter  N=double(2)  Nmax=16  RateOptions=Allow multirate processing  ic=0  mode=Unused parameter value
  in3_repeat : dspsigops/Repeat  FactorSource=Dialog parameter  N=double(2)  Nmax=16  RateOptions=Allow multirate processing  ic=0  mode=Unused parameter value
  in3_repeat1 : dspsigops/Repeat  FactorSource=Dialog parameter  N=double(2)  Nmax=16  RateOptions=Allow multirate processing  ic=0  mode=Unused parameter value
  in3_repeat2 : dspsigops/Repeat  FactorSource=Dialog parameter  N=double(2)  Nmax=16  RateOptions=Allow multirate processing  ic=0  mode=Unused parameter value
  in4_repeat : dspsigops/Repeat  FactorSource=Dialog parameter  N=double(2)  Nmax=16  RateOptions=Allow multirate processing  ic=0  mode=Unused parameter value
  in4_repeat1 : dspsigops/Repeat  FactorSource=Dialog parameter  N=double(2)  Nmax=16  RateOptions=Allow multirate processing  ic=0  mode=Unused parameter value
  in4_repeat2 : dspsigops/Repeat  FactorSource=Dialog parameter  N=double(2)  Nmax=16  RateOptions=Allow multirate processing  ic=0  mode=Unused parameter value
  in5_repeat : dspsigops/Repeat  FactorSource=Dialog parameter  N=double(2)  Nmax=16  RateOptions=Allow multirate processing  ic=0  mode=Unused parameter value
  in6_repeat : dspsigops/Repeat  FactorSource=Dialog parameter  N=double(2)  Nmax=16  RateOptions=Allow multirate processing  ic=0  mode=Unused parameter value
  rd_{0..2,4..5,11..12,21..22,41..42,51..52} (13 alike) : Delay  DelayLength=double(1)  InitialCondition=0
  rd_01 : Delay  DelayLength=double(1)  InitialCondition=0
  rd_02 : Delay  DelayLength=double(1)  InitialCondition=0
  rd_6 : Delay  DelayLength=double(2)  InitialCondition=0
  rotate : Subsystem
  data_out : Outport  SampleTime=2e-08  InitialOutput=0
  valid_out : Outport  Port=2  SampleTime=2e-08  InitialOutput=0
  wires:
  data_in/1 -> in3_repeat/1
  valid_in/1 -> in0_repeat/1
  s1_in/1 -> in5_repeat/1
  s2_in/1 -> in4_repeat/1
  Delay2_absorbed/1 -> data_out/1, in3_repeat2/1
  Enable_out9/1 -> in1_repeat/1, in1_repeat1/1, in1_repeat2/1
  Delay3_absorbed/1 -> valid_out/1, in2_repeat/1
  in0_repeat/1 -> rd_0/1
  in1_repeat/1 -> rd_1/1
  in4_repeat/1 -> rotate/1(s2)
  in5_repeat/1 -> rotate/2(s1)
  in1_repeat1/1 -> rd_11/1
  in3_repeat/1 -> rd_41/1
  in1_repeat2/1 -> rd_12/1
  in4_repeat1/1 -> rd_52/1
  in3_repeat1/1 -> rd_42/1
  in2_repeat/1 -> rd_22/1
  Delay/1 -> Delay_absorbed/1
  Delay_absorbed/1 -> in4_repeat2/1, in3_repeat1/1
  in4_repeat2/1 -> rd_51/1
  in2_repeat1/1 -> rd_21/1
  Delay1/1 -> Delay_absorbed1/1
  Delay_absorbed1/1 -> in6_repeat/1, in4_repeat1/1
  in6_repeat/1 -> rotate/3(data_in)
  Delay2/1 -> Delay2_absorbed/1
  in3_repeat2/1 -> rd_6/1
  in2_repeat2/1 -> rd_2/1
  crp_out_delay/1 -> Delay11/1
  Delay2_enbsw/1 -> Delay2/1
  Delay11/1 -> Delay1_absorbed/1
  Delay1_absorbed/1 -> in2_repeat2/1, in0_repeat1/1
  in0_repeat1/1 -> rd_01/1
  crp_out_delay1/1 -> Delay12/1
  crp_out_delay2/1 -> Delay/1
  Delay12/1 -> Delay1_absorbed1/1
  Delay1_absorbed1/1 -> in2_repeat1/1, in0_repeat2/1
  in0_repeat2/1 -> rd_02/1
  crp_out_delay3/1 -> Delay3/1
  crp_out_delay4/1 -> Delay1/1
  Delay3/1 -> Delay3_absorbed/1
  Delay1_enbsw/1 -> crp_out_delay/1
  rotate/1(data_out) -> rd_4/1
  rd_6/1 -> Delay2_enbsw/3
  rd_0/1 -> Delay1_enbsw/1
  rd_2/1 -> Delay1_enbsw/3
  rd_4/1 -> Delay2_enbsw/1
  rd_1/1 -> Delay1_enbsw/2, rd_5/1
  rd_5/1 -> Delay2_enbsw/2
  Delay1_enbsw1/1 -> crp_out_delay1/1
  Delay_enbsw/1 -> crp_out_delay2/1
  rd_41/1 -> Delay_enbsw/1
  rd_51/1 -> Delay_enbsw/3
  rd_01/1 -> Delay1_enbsw1/1
  rd_21/1 -> Delay1_enbsw1/3
  rd_11/1 -> Delay1_enbsw1/2, Delay_enbsw/2
  Delay3_enbsw/1 -> crp_out_delay3/1
  Delay_enbsw1/1 -> crp_out_delay4/1
  rd_42/1 -> Delay_enbsw1/1
  rd_52/1 -> Delay_enbsw1/3
  rd_02/1 -> Delay3_enbsw/1
  rd_22/1 -> Delay3_enbsw/3
  rd_12/1 -> Delay3_enbsw/2, Delay_enbsw1/2

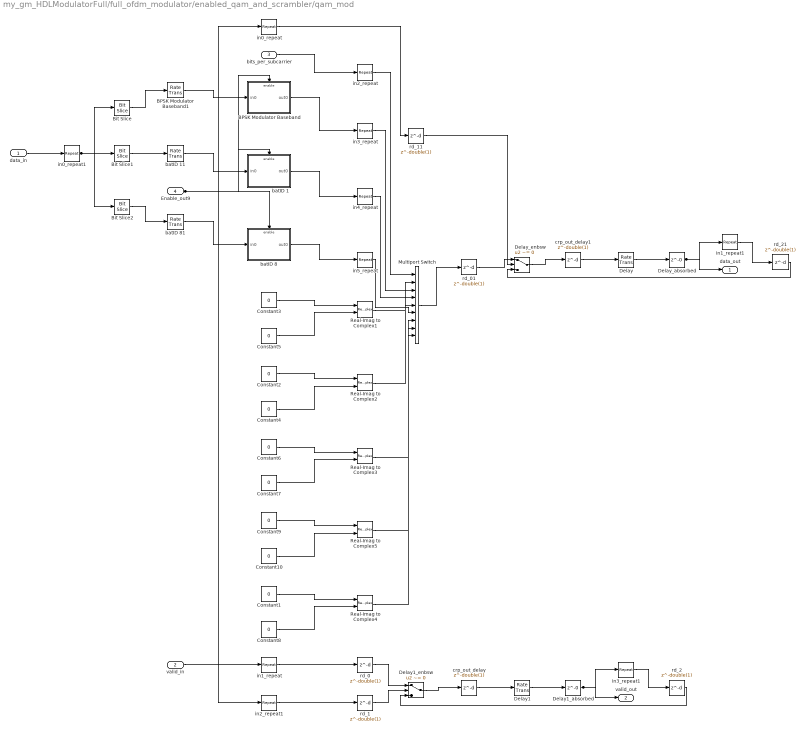
== system my_gm_HDLModulatorFull/full_ofdm_modulator/enabled_qam_and_scrambler/qam_mod ==
  data_in : Inport  OutDataTypeStr=fixdt(0, 12, 0)  SampleTime=2e-08
  valid_in : Inport  Port=2  OutDataTypeStr=boolean  SampleTime=2e-08
  bits_per_subcarrier : Inport  Port=3  OutDataTypeStr=fixdt(0, 4, 0)  SampleTime=2e-08
  Enable_out9 : Inport  Port=4  OutDataTypeStr=boolean  SampleTime=2e-08
  BPSK Modulator Baseband : Subsystem
      settings: MinAlgLoopOccurrences=on
  BPSK Modulator Baseband1 : RateTransition  OutPortSampleTimeOpt=Multiple of input port sample time  OutPortSampleTimeMultiple=2
  Bit Slice : hdlsllib/Logic and Bit Operations/Bit Slice  lidx=double(0)  ridx=double(0)
  Bit Slice1 : hdlsllib/Logic and Bit Operations/Bit Slice  lidx=double(1)  ridx=double(0)
  Bit Slice2 : hdlsllib/Logic and Bit Operations/Bit Slice  lidx=double(3)  ridx=double(0)
  Constant{1..10} (10 alike) : Constant  Value=0  OutDataTypeStr=fixdt(1, 16, 14)  SampleTime=1e-08
  Delay : RateTransition  OutPortSampleTimeOpt=Multiple of input port sample time  OutPortSampleTimeMultiple=2
  Delay1 : RateTransition  OutPortSampleTimeOpt=Multiple of input port sample time  OutPortSampleTimeMultiple=2
  Delay1_absorbed : Delay  DelayLength=0
  Delay1_enbsw : Switch  Criteria=u2 ~= 0  Threshold=double(0)  OutDataTypeStr=boolean  SampleTime=1e-08  SaturateOnIntegerOverflow=off  InputSameDT=off
  Delay_absorbed : Delay  DelayLength=0
  Delay_enbsw : Switch  Criteria=u2 ~= 0  Threshold=double(0)  OutDataTypeStr=fixdt(1, 16, 14)  SampleTime=1e-08  SaturateOnIntegerOverflow=off  InputSameDT=off
  Multiport Switch : MultiPortSwitch  DataPortOrder=Zero-based contiguous  Inputs=8  DiagnosticForDefault=None  zeroidx=on  OutDataTypeStr=fixdt(1, 16, 14)  SampleTime=1e-08  SaturateOnIntegerOverflow=off  InputSameDT=off
  Real-Imag to Complex{1..5} (5 alike) : RealImagToComplex  ConstantPart="fi(0,1,16,14,\"hex\",\"0000\")"  SampleTime=1e-08
  batID 1 : Subsystem
      settings: MinAlgLoopOccurrences=on
  batID 11 : RateTransition  OutPortSampleTimeOpt=Multiple of input port sample time  OutPortSampleTimeMultiple=2
  batID 8 : Subsystem
      settings: MinAlgLoopOccurrences=on
  batID 81 : RateTransition  OutPortSampleTimeOpt=Multiple of input port sample time  OutPortSampleTimeMultiple=2
  crp_out_delay : Delay  DelayLength=double(1)  InitialCondition=0
  crp_out_delay1 : Delay  DelayLength=double(1)  InitialCondition=0
  in0_repeat : dspsigops/Repeat  FactorSource=Dialog parameter  N=double(2)  Nmax=16  RateOptions=Allow multirate processing  ic=0  mode=Unused parameter value
  in0_repeat1 : dspsigops/Repeat  FactorSource=Dialog parameter  N=double(2)  Nmax=16  RateOptions=Allow multirate processing  ic=0  mode=Unused parameter value
  in1_repeat : dspsigops/Repeat  FactorSource=Dialog parameter  N=double(2)  Nmax=16  RateOptions=Allow multirate processing  ic=0  mode=Unused parameter value
  in1_repeat1 : dspsigops/Repeat  FactorSource=Dialog parameter  N=double(2)  Nmax=16  RateOptions=Allow multirate processing  ic=0  mode=Unused parameter value
  in2_repeat : dspsigops/Repeat  FactorSource=Dialog parameter  N=double(2)  Nmax=16  RateOptions=Allow multirate processing  ic=0  mode=Unused parameter value
  in2_repeat1 : dspsigops/Repeat  FactorSource=Dialog parameter  N=double(2)  Nmax=16  RateOptions=Allow multirate processing  ic=0  mode=Unused parameter value
  in3_repeat : dspsigops/Repeat  FactorSource=Dialog parameter  N=double(2)  Nmax=16  RateOptions=Allow multirate processing  ic=0  mode=Unused parameter value
  in3_repeat1 : dspsigops/Repeat  FactorSource=Dialog parameter  N=double(2)  Nmax=16  RateOptions=Allow multirate processing  ic=0  mode=Unused parameter value
  in4_repeat : dspsigops/Repeat  FactorSource=Dialog parameter  N=double(2)  Nmax=16  RateOptions=Allow multirate processing  ic=0  mode=Unused parameter value
  in5_repeat : dspsigops/Repeat  FactorSource=Dialog parameter  N=double(2)  Nmax=16  RateOptions=Allow multirate processing  ic=0  mode=Unused parameter value
  rd_{0..2,11,21} (5 alike) : Delay  DelayLength=double(1)  InitialCondition=0
  rd_01 : Delay  DelayLength=double(1)  InitialCondition=0
  data_out : Outport  SampleTime=2e-08  InitialOutput=0
  valid_out : Outport  Port=2  SampleTime=2e-08  InitialOutput=0
  wires:
  data_in/1 -> in0_repeat1/1
  valid_in/1 -> in1_repeat/1
  bits_per_subcarrier/1 -> in2_repeat/1
  BPSK Modulator Baseband/1(out0) -> in3_repeat/1
  BPSK Modulator Baseband1/1 -> BPSK Modulator Baseband/1(in0)
  batID 11/1 -> batID 1/1(in0)
  batID 81/1 -> batID 8/1(in0)
  batID 1/1(out0) -> in4_repeat/1
  batID 8/1(out0) -> in5_repeat/1
  Enable_out9/1 -> batID 8/Enable, batID 1/Enable, BPSK Modulator Baseband/Enable, in0_repeat/1, in2_repeat1/1
  Delay_absorbed/1 -> data_out/1, in1_repeat1/1
  Delay1_absorbed/1 -> valid_out/1, in3_repeat1/1
  in0_repeat/1 -> rd_11/1
  in2_repeat/1 -> Multiport Switch/1
  in3_repeat/1 -> Multiport Switch/3
  in4_repeat/1 -> Multiport Switch/4
  in5_repeat/1 -> Multiport Switch/6
  in0_repeat1/1 -> Bit Slice/1, Bit Slice2/1, Bit Slice1/1
  in1_repeat/1 -> rd_0/1
  in2_repeat1/1 -> rd_1/1
  Bit Slice1/1 -> batID 11/1
  Bit Slice2/1 -> batID 81/1
  Bit Slice/1 -> BPSK Modulator Baseband1/1
  in3_repeat1/1 -> rd_2/1
  crp_out_delay/1 -> Delay1/1
  Delay1/1 -> Delay1_absorbed/1
  in1_repeat1/1 -> rd_21/1
  crp_out_delay1/1 -> Delay/1
  Delay/1 -> Delay_absorbed/1
  Delay1_enbsw/1 -> crp_out_delay/1
  rd_0/1 -> Delay1_enbsw/1
  rd_1/1 -> Delay1_enbsw/2
  rd_2/1 -> Delay1_enbsw/3
  Delay_enbsw/1 -> crp_out_delay1/1
  Constant3/1 -> Real-Imag to Complex1/1
  Constant5/1 -> Real-Imag to Complex1/2
  Real-Imag to Complex1/1 -> Multiport Switch/2
  Constant2/1 -> Real-Imag to Complex2/1
  Constant4/1 -> Real-Imag to Complex2/2
  Real-Imag to Complex2/1 -> Multiport Switch/5
  Constant6/1 -> Real-Imag to Complex3/1
  Constant7/1 -> Real-Imag to Complex3/2
  Real-Imag to Complex3/1 -> Multiport Switch/7
  Constant9/1 -> Real-Imag to Complex5/1
  Constant10/1 -> Real-Imag to Complex5/2
  Real-Imag to Complex5/1 -> Multiport Switch/8
  Constant1/1 -> Real-Imag to Complex4/1
  Constant8/1 -> Real-Imag to Complex4/2
  Real-Imag to Complex4/1 -> Multiport Switch/9
  Multiport Switch/1 -> rd_01/1
  rd_11/1 -> Delay_enbsw/2
  rd_21/1 -> Delay_enbsw/3
  rd_01/1 -> Delay_enbsw/1

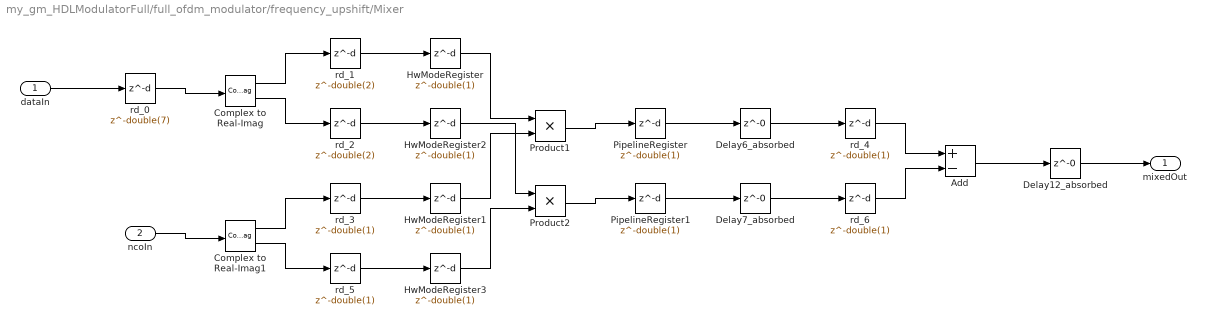
== system my_gm_HDLModulatorFull/full_ofdm_modulator/frequency_upshift/Mixer ==
  dataIn : Inport  OutDataTypeStr=fixdt(1, 16, 14)  PortDimensions=1  SampleTime=1e-08
      settings: SignalType=complex
  ncoIn : Inport  Port=2  OutDataTypeStr=fixdt(1, 16, 14)  PortDimensions=1  SampleTime=1e-08
      settings: SignalType=complex
  Add : Sum  Inputs=+-  OutDataTypeStr=fixdt(1, 16, 14)  AccumDataTypeStr=fixdt(1, 16, 14)  SampleTime=1e-08
  Complex to Real-Imag : ComplexToRealImag  SampleTime=1e-08
  Complex to Real-Imag1 : ComplexToRealImag  SampleTime=1e-08
  Delay12_absorbed : Delay  DelayLength=0
  Delay6_absorbed : Delay  DelayLength=0
  Delay7_absorbed : Delay  DelayLength=0
  HwModeRegister{,1..3} (4 alike) : Delay  DelayLength=double(1)  InitialCondition=0  SampleTime=1e-08
  PipelineRegister : Delay  DelayLength=double(1)  InitialCondition=0  SampleTime=1e-08
  PipelineRegister1 : Delay  DelayLength=double(1)  InitialCondition=0  SampleTime=1e-08
  Product1 : Product  Inputs=**  OutDataTypeStr=fixdt(1, 16, 14)  SampleTime=1e-08
  Product2 : Product  Inputs=**  OutDataTypeStr=fixdt(1, 16, 14)  SampleTime=1e-08
  rd_0 : Delay  DelayLength=double(7)  InitialCondition=0  SampleTime=1e-08
  rd_1 : Delay  DelayLength=double(2)  InitialCondition=0  SampleTime=1e-08
  rd_2 : Delay  DelayLength=double(2)  InitialCondition=0  SampleTime=1e-08
  rd_{3..6} (4 alike) : Delay  DelayLength=double(1)  InitialCondition=0  SampleTime=1e-08
  mixedOut : Outport  SampleTime=1e-08
  wires:
  dataIn/1 -> rd_0/1
  ncoIn/1 -> Complex to Real-Imag1/1
  Add/1 -> Delay12_absorbed/1
  Complex to Real-Imag/1 -> rd_1/1
  Complex to Real-Imag/2 -> rd_2/1
  Complex to Real-Imag1/1 -> rd_3/1
  Complex to Real-Imag1/2 -> rd_5/1
  Delay12_absorbed/1 -> mixedOut/1
  Delay6_absorbed/1 -> rd_4/1
  Delay7_absorbed/1 -> rd_6/1
  PipelineRegister/1 -> Delay6_absorbed/1
  PipelineRegister1/1 -> Delay7_absorbed/1
  rd_0/1 -> Complex to Real-Imag/1
  rd_1/1 -> HwModeRegister/1
  rd_2/1 -> HwModeRegister2/1
  rd_3/1 -> HwModeRegister1/1
  rd_5/1 -> HwModeRegister3/1
  rd_6/1 -> Add/2
  rd_4/1 -> Add/1
  Product1/1 -> PipelineRegister/1
  HwModeRegister/1 -> Product1/1
  HwModeRegister1/1 -> Product1/2
  Product2/1 -> PipelineRegister1/1
  HwModeRegister2/1 -> Product2/1
  HwModeRegister3/1 -> Product2/2

== system my_gm_HDLModulatorFull/full_ofdm_modulator/interpolator/falling_edge_detector ==
  in : Inport  OutDataTypeStr=boolean  SampleTime=1e-08
  Delay : Delay  DelayLength=double(1)  InitialCondition=0  SampleTime=1e-08
  Logical Operator : Logic  AllPortsSameDT=off  OutDataTypeStr=boolean  SampleTime=1e-08
  Logical Operator1 : Logic  Operator=NOT  Inputs=1  AllPortsSameDT=off  OutDataTypeStr=boolean  SampleTime=1e-08
  out : Outport  SampleTime=1e-08
  wires:
  in/1 -> Logical Operator1/1, Delay/1
  Delay/1 -> Logical Operator/2
  Logical Operator/1 -> out/1
  Logical Operator1/1 -> Logical Operator/1
